simulink model "InverseKinematics_DirectionalController2018b"  (R2018b)
settings: Solver=VariableStepAuto  StartTime=0.0  StopTime=inf  RelTol=1e-3
undefined symbols (not defined in the file): f
libraries: instrumentlib x15, dspnetwork x6
(part 3 of 3)

== matlab function InverseKinematics_DirectionalController2018b/MATLAB Function4 ==
  data: u input; y output
function y = fcn(u)

if u > 1
    c = sprintf('%f', u);
    y = str2double(c(2:6));
    disp(y);
else
    y = u;
end

== matlab function InverseKinematics_DirectionalController2018b/MATLAB Function5 ==
  data: u input; y output; x input; z input
function y = fcn(u, x, z)

if z == 1
    if u < 1
        %c = sprintf('%f', u);
        y = x + u;
        disp(y);
    else
        y = u;
    end
else
    y = u;
end

== matlab function InverseKinematics_DirectionalController2018b/MATLAB Function6 ==
  data: u input; y output; x input; z input
function y = fcn(u, x, z)

if z == 1
    if u < 1
        %c = sprintf('%f', u);
        y = x + u;
        disp(y);
    else
        y = u;
    end
else
    y = u;
end

== matlab function InverseKinematics_DirectionalController2018b/MATLAB Function7 ==
  data: u input; y output
function y = fcn(u)

%x = [u(1); -u(2); u(3)];
%y = x/29;

%
%y = zeros(length(u));

y = [0,0,0,0,0,0];

for i = 1:length(u)
    if u(i) < 0
        y(i) = u(i) + 2*pi;
    else
        y(i) = u(i);
    end
end

== matlab function InverseKinematics_DirectionalController2018b/MATLAB Function8 ==
  data: u input; y output
function y = fcn(u)

x = [u(1); u(2); u(3)];
y = x/29;
